simulink model "dcmotor"  (Simulink 8.9)
settings: Solver=ode45  StartTime=0.0  StopTime=1  RelTol=1e-9  EnableMultiTasking=on
values from neighbouring files (symbols this model uses):
  B = 0.000979532163743    [matlab.mat]    (also in mopar.m)
  J = 3.35e-06    [matlab.mat]    (also in mopar.m)
  K_T = 0.0139    [matlab.mat]    (also in mopar.m)
  K_v = 0.013940578957    [matlab.mat]    (also in mopar.m)
  Kp = 100    [matlab.mat]    (also in motor.m)
  L_a = 3.45e-05    [matlab.mat]    (also in mopar.m)
  R_a = 0.198    [matlab.mat]    (also in mopar.m)
  Td = 0.00117375026294    [matlab.mat]    (also in motor.m = 0.19/(W_c*sqrt(a)))
settings Model: SuppressorTable=22 serialization::archive 11 0 6 0 0 0 0 0  Creator=thomakro  LastModifiedBy=erlingtveter
settings OptimizationCC: ExpressionDepthLimit=2147483647  InitFltsAndDblsToZero=on
settings DebuggingCC: SaveWithParameterizedLinksMsg=none  SignalResolutionControl=TryResolveAllWithWarning  SolverPrmCheckMsg=warning
settings GRTTargetCC: TargetFcnLib=ansi_tfl_tmw.mat

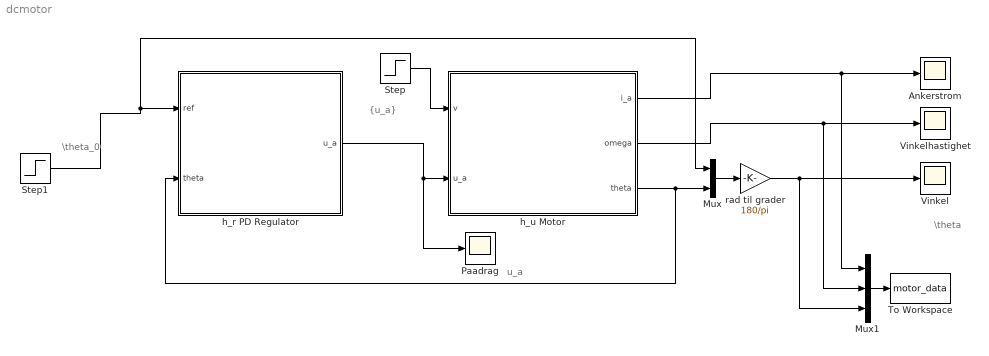
== system dcmotor ==
  note: {u_a}
  note: \theta
  note: \theta_0
  note: u_a
  Ankerstrom : Scope
  Mux : Mux  Inputs=2
  Mux1 : Mux  Inputs=3
  Paadrag : Scope
  Step : Step  Time=0.2  SampleTime=0
  Step1 : Step  Time=0  SampleTime=0
  To Workspace : ToWorkspace  VariableName=motor_data  SaveFormat=Structure With Time  SampleTime=-1
  Vinkel : Scope
  Vinkelhastighet : Scope
  h_r PD Regulator : Subsystem  mask{Kp=Kp, Td=Td}
      mask Display:
      | image(imread('maxon_ctrl.jpg'))
      | port_label('input',1,'ref','texmode','on')
      | port_label('input',2,'\theta','texmode','on')
      | port_label('output',1,'u_a','texmode','on')
  h_u Motor : Subsystem
      mask Display:
      | image(imread('maxon_dc.jpg'));
      | disp('DC Motor')
      | port_label('output',1,'i_a','texmode','on')
      | port_label('output',2,'\omega','texmode','on')
      | port_label('output',3,'\theta','texmode','on')
      | port_label('input',1,'v','texmode','on')
      | port_label('input',2,'u_a','texmode','on')
  rad til grader : Gain  Gain=180/pi
  wires:
  h_u Motor/3(theta) -> h_r PD Regulator/2(theta), Mux/2
  Mux/1 -> rad til grader/1
  rad til grader/1 -> Mux1/3, Vinkel/1
  h_u Motor/2(omega) -> Mux1/2, Vinkelhastighet/1
  h_u Motor/1(i_a) -> Mux1/1, Ankerstrom/1
  Step1/1 -> h_r PD Regulator/1(ref), Mux/1
  Mux1/1 -> To Workspace/1
  h_r PD Regulator/1(u_a) -> Paadrag/1, h_u Motor/2(u_a)
  Step/1 -> h_u Motor/1(v)

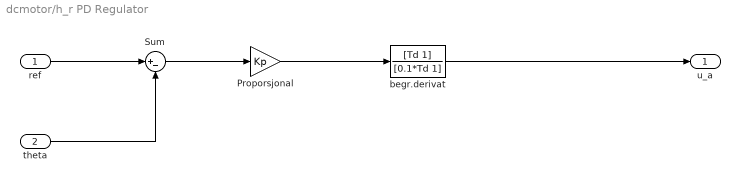
== system dcmotor/h_r PD Regulator ==
  ref : Inport
  theta : Inport  Port=2
  Proporsjonal : Gain  Gain=Kp
  Sum : Sum  Inputs=|+-
  begr.derivat : TransferFcn  Numerator=[Td 1]  Denominator=[0.1*Td 1]
  u_a : Outport
  wires:
  Sum/1 -> Proporsjonal/1
  theta/1 -> Sum/2
  ref/1 -> Sum/1
  begr.derivat/1 -> u_a/1
  Proporsjonal/1 -> begr.derivat/1

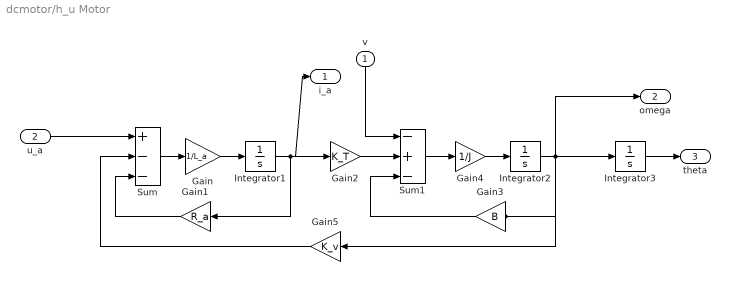
== system dcmotor/h_u Motor ==
  v : Inport
  u_a : Inport  Port=2
  Gain : Gain  Gain=1/L_a  SaturateOnIntegerOverflow=on  OutDataTypeStr=Inherit: Same as input  ParamDataTypeStr=Inherit: Same as input
  Gain1 : Gain  Gain=R_a  SaturateOnIntegerOverflow=on  OutDataTypeStr=Inherit: Same as input  ParamDataTypeStr=Inherit: Same as input
  Gain2 : Gain  Gain=K_T  SaturateOnIntegerOverflow=on  OutDataTypeStr=Inherit: Same as input  ParamDataTypeStr=Inherit: Same as input
  Gain3 : Gain  Gain=B  SaturateOnIntegerOverflow=on  OutDataTypeStr=Inherit: Same as input  ParamDataTypeStr=Inherit: Same as input
  Gain4 : Gain  Gain=1/J  SaturateOnIntegerOverflow=on  OutDataTypeStr=Inherit: Same as input  ParamDataTypeStr=Inherit: Same as input
  Gain5 : Gain  Gain=K_v  SaturateOnIntegerOverflow=on  OutDataTypeStr=Inherit: Same as input  ParamDataTypeStr=Inherit: Same as input
  Integrator1 : Integrator  UpperSaturationLimit=4  LowerSaturationLimit=-4
  Integrator2 : Integrator
  Integrator3 : Integrator
  Sum : Sum  Inputs=+--  SaturateOnIntegerOverflow=on  InputSameDT=on  OutDataTypeStr=Inherit: Same as first input
  Sum1 : Sum  Inputs=-+-  SaturateOnIntegerOverflow=on  InputSameDT=on  OutDataTypeStr=Inherit: Same as first input
  i_a : Outport  InitialOutput=0
  omega : Outport  Port=2  InitialOutput=0
  theta : Outport  Port=3  InitialOutput=0
  wires:
  Sum/1 -> Gain/1
  Gain2/1 -> Sum1/2
  Gain3/1 -> Sum1/3
  v/1 -> Sum1/1
  Gain/1 -> Integrator1/1
  Integrator1/1 -> Gain2/1, Gain1/1, i_a/1
  Sum1/1 -> Gain4/1
  Gain4/1 -> Integrator2/1
  Integrator2/1 -> Gain3/1, Gain5/1, omega/1, Integrator3/1
  Integrator3/1 -> theta/1
  Gain1/1 -> Sum/3
  Gain5/1 -> Sum/2
  u_a/1 -> Sum/1
